simulink model "sf_nest"  (R2015b)
settings: Solver=FixedStepDiscrete  SolverMode=SingleTasking  StartTime=0.0  StopTime=2/10  RelTol=1e-3
settings Model: Creator=at-mt  LastModifiedBy=amatsumo
settings DataIOCC: SaveFormat=Array  SignalLoggingSaveFormat=ModelDataLogs  SaveOutput=off  SignalLogging=off  SaveTime=off
settings OptimizationCC: BlockReduction=off  ConditionallyExecuteInputs=off  DefaultParameterBehavior=Inlined  ExpressionDepthLimit=2147483647
settings DebuggingCC: AlgebraicLoopMsg=error  UnderspecifiedInitializationDetection=Classic  MergeDetectMultiDrivingBlocksExec=none  SolverPrmCheckMsg=warning  SingleTaskRateTransMsg=error  FcnCallInpInsideContextMsg=UseLocalSettings  StateNameClashWarn=warning
settings HardwareCC: ProdBitPerPointer=32  ProdLargestAtomicFloat=None  ProdIntDivRoundTo=Undefined  ProdEndianess=Unspecified  ProdWordSize=32  ProdHWDeviceType=ASIC/FPGA->ASIC/FPGA  ProdEqTarget=off
settings GRTTargetCC: GeneratePreprocessorConditionals=Disable all  CombineOutputUpdateFcns=off  GRTInterface=on
settings ConfigComp: CovMetricSettings=dcmw  CovHTMLOptions=-aTS=1 -bRG=1 -bTC=1 -hTR=0 -nFC=0 -scm=1 -bcm=1 -xEv=0  CovSFcnEnable=off

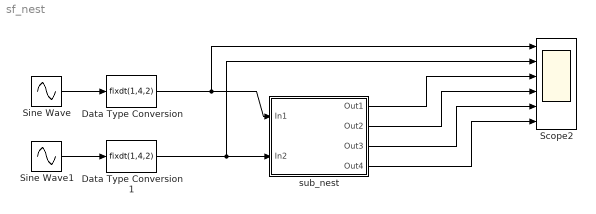
== system sf_nest ==
  Data Type Conversion : DataTypeConversion  OutDataTypeStr=fixdt(1,4,2)
  Data Type Conversion1 : DataTypeConversion  OutDataTypeStr=fixdt(1,4,2)
  Scope2 : Scope  NumInputPorts=6
  Sine Wave : Sin  Amplitude=4  Frequency=2*pi*10  SampleTime=1/100
  Sine Wave1 : Sin  Amplitude=4  Frequency=2*pi*20  SampleTime=1/100
  sub_nest : Subsystem
  wires:
  Sine Wave/1 -> Data Type Conversion/1
  Data Type Conversion/1 -> sub_nest/1(In1), Scope2/1
  Sine Wave1/1 -> Data Type Conversion1/1
  Data Type Conversion1/1 -> sub_nest/2(In2), Scope2/2
  sub_nest/1(Out1) -> Scope2/3
  sub_nest/2(Out2) -> Scope2/4
  sub_nest/3(Out3) -> Scope2/5
  sub_nest/4(Out4) -> Scope2/6

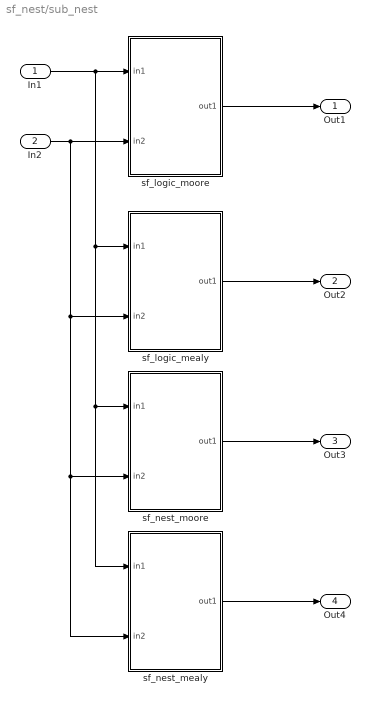
== system sf_nest/sub_nest ==
  In1 : Inport
  In2 : Inport  Port=2
  sf_logic_mealy : Stateflow chart  TreatAsAtomicUnit=on
  sf_logic_moore : Stateflow chart  TreatAsAtomicUnit=on
  sf_nest_mealy : Stateflow chart  TreatAsAtomicUnit=on
  sf_nest_moore : Stateflow chart  TreatAsAtomicUnit=on
  Out1 : Outport
  Out2 : Outport  Port=2
  Out3 : Outport  Port=3
  Out4 : Outport  Port=4
  wires:
  sf_logic_moore/1(out1) -> Out1/1
  sf_logic_mealy/1(out1) -> Out2/1
  sf_nest_mealy/1(out1) -> Out4/1
  sf_nest_moore/1(out1) -> Out3/1
  In1/1 -> sf_logic_moore/1(in1), sf_logic_mealy/1(in1), sf_nest_moore/1(in1), sf_nest_mealy/1(in1)
  In2/1 -> sf_logic_moore/2(in2), sf_logic_mealy/2(in2), sf_nest_moore/2(in2), sf_nest_mealy/2(in2)

== stateflow chart sf_nest/sub_nest/sf_logic_moore ==
  settings: updateMethod=DISCRETE  stateMachineType=MOORE_MACHINE  executeAtInitialization=1  initializeOutput=1
  state Init/
    out1 = 2;
  state On1/
    out1 = 1;
  Init -> Init [order 2]
  (default) -> Init
  Init -> On1 [order 1] : [(in1 < 0)&&(in2<0)]
  On1 -> Init [order 1] : [(in1>=0)&&(in2>=0)]
  On1 -> On1 [order 2]
  data: in1 input fixdt(1,4,2) size=1; out1 output fixdt(0,4,0); in2 input fixdt(1,4,2)

== stateflow chart sf_nest/sub_nest/sf_nest_moore ==
  settings: updateMethod=DISCRETE  stateMachineType=MOORE_MACHINE  executeAtInitialization=1  initializeOutput=1
  state Init/
    out1 = 2;
  state On1/
    out1 = 1;
  Init -> Init [order 2]
  (default) -> Init
  Init -> (junction 59) [order 1] : [(in1<0)]
  (junction 59) -> Init [order 2]
  (junction 62) -> Init [order 1] : [(in2>=0)]
  (junction 62) -> On1 [order 2]
  On1 -> (junction 62) [order 1] : [(in1>=0)]
  (junction 59) -> On1 [order 1] : [(in2<0)]
  On1 -> On1 [order 2]
  data: in1 input fixdt(1,4,2) size=1; out1 output fixdt(0,4,0); in2 input fixdt(1,4,2)

== stateflow chart sf_nest/sub_nest/sf_logic_mealy ==
  settings: updateMethod=DISCRETE  stateMachineType=MEALY_MACHINE  executeAtInitialization=1  initializeOutput=1
  state Init/
  state On1/
  Init -> Init [order 2] : {out1 = 2;}
  (default) -> Init
  Init -> On1 [order 1] : [(in1 < 0)&&(in2<0)]
      | {out1 = 1;}
  On1 -> Init [order 1] : [(in1>=0)&&(in2>=0)]
      | {out1 = 2;}
  On1 -> On1 [order 2] : {out1 = 1;}
  data: in1 input fixdt(1,4,2) size=1; out1 output fixdt(0,4,0); in2 input fixdt(1,4,2)

== stateflow chart sf_nest/sub_nest/sf_nest_mealy ==
  settings: updateMethod=DISCRETE  stateMachineType=MEALY_MACHINE  executeAtInitialization=1  initializeOutput=1
  state Init/
  state On1/
  Init -> Init [order 2] : //[in >=0]
      | {out1 = 2;}
  (default) -> Init
  Init -> (junction 58) [order 1] : [(in1 < 0)]
  (junction 58) -> Init [order 2] : {out1 = 2;}
  (junction 61) -> Init [order 1] : [(in2>=0)]
      | {out1 = 2;}
  (junction 58) -> On1 [order 1] : [(in2<0)]
      | {out1 = 1;}
  (junction 61) -> On1 [order 2] : {out1 = 1;}
  On1 -> (junction 61) [order 1] : [(in1>=0)]
  On1 -> On1 [order 2] : //[in < 0]
      | {out1 = 1;}
  data: in1 input fixdt(1,4,2) size=1; out1 output fixdt(0,4,0); in2 input fixdt(1,4,2)
